simulink model "robotarm_NN"  (R2018b)
settings: Solver=FixedStepAuto  StartTime=0.0  StopTime=20  RelTol=1e-3  AbsTol=1e-6
undefined symbols (not defined in the file or in its folder): options
libraries: neural x132, simulink x2
(part 2 of 6)

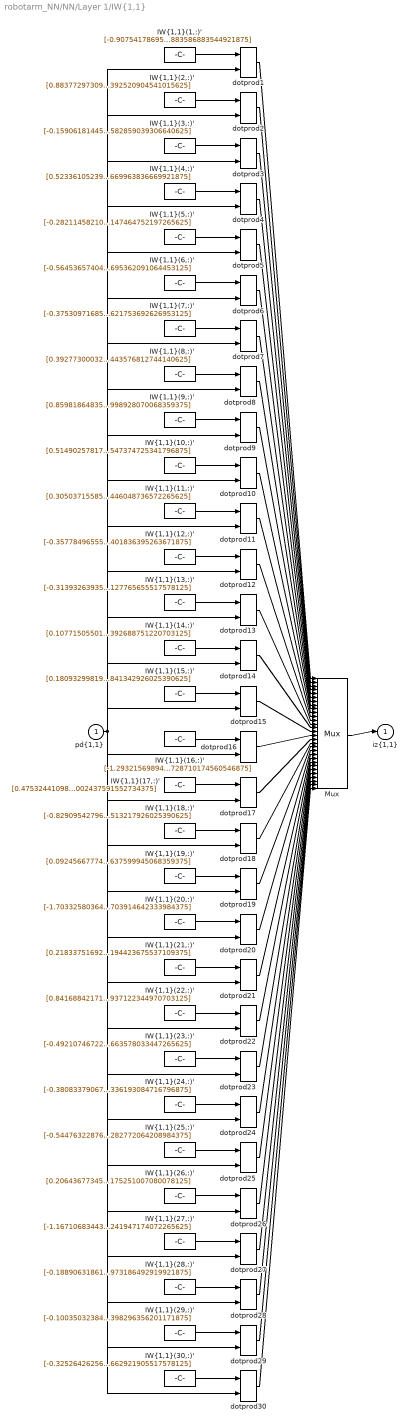
== system robotarm_NN/NN/Layer 1/IW{1,1} ==
  "pd{1,1}" : Inport  PortDimensions=10
      mask Display: e = 0.06;c1 = [120 230 180]/255;c2 = ([120 230 180]+0)/(256+128);c3 = ([120 230 180]+128)/(256+128);patch([0 1 1 0],[0 0 1 1],c1);patch([0 1 1 1-e 1-e 0+e],[0 0 1 1-e 0+e 0+e],c2);patch([0 0 1 1-e 0+e 0+e],[0 1 1 1-e 1-e 0+e],c3);plot([0 1 1 0 0],[0 0 1 1 0]);
  "IW{1,1}(1,:)'" : Constant  Value=[-0.90754178695281095823332861982635222375392913818359375;-0.742116818964511981704390564118511974811553955078125;0.412008312868980153265141552765271626412868499755859375;0.36505650495964692137107476810342632234096527099609375;0.8146542718376459379925336179439909756183624267578125;0.74217006261127071997663051661220379173755645751953125;-0.61338539843698958176076985182589851319789886474609375;-0.7369042666159348886623092766967602074146270751953125;0.67520008036012690855187656779889948666095733642578125;0.66999644798205515439093460372532717883586883544921875]
      mask Display: e = 0.06;c1 = [120 150 230]/255;c2 = ([120 150 230]+0)/383;c3 = ([120 150 230]+128)/383;patch([0 1 1 0],[0 0 1 1],c1);patch([0 1 1 1-e 1-e 0+e],[0 0 1 1-e 0+e 0+e],c2);patch([0 0 1 1-e 0+e 0+e],[0 1 1 1-e 1-e 0+e],c3);plot([0 1 1 0 0],[0 0 1 1 0]);disp('Weights');
  "IW{1,1}(10,:)'" : Constant  Value=[0.51490257817894524716706428080215118825435638427734375;-0.55689013510191454070508143558981828391551971435546875;-1.0160440906229057933529702495434321463108062744140625;0.833148456201297182843745758873410522937774658203125;0.2978923037071978807688310553203336894512176513671875;0.44937108713853712860242239912622608244419097900390625;-1.232430563498764453100875471136532723903656005859375;0.51275755356745766899706495678401552140712738037109375;0.271725160862764714142514321792987175285816192626953125;-0.256572494217802204996559112260001711547374725341796875]
      mask Display: e = 0.06;c1 = [120 150 230]/255;c2 = ([120 150 230]+0)/383;c3 = ([120 150 230]+128)/383;patch([0 1 1 0],[0 0 1 1],c1);patch([0 1 1 1-e 1-e 0+e],[0 0 1 1-e 0+e 0+e],c2);patch([0 0 1 1-e 0+e 0+e],[0 1 1 1-e 1-e 0+e],c3);plot([0 1 1 0 0],[0 0 1 1 0]);disp('Weights');
  "IW{1,1}(11,:)'" : Constant  Value=[0.305037155853193298060688221085001714527606964111328125;-0.2027495084904122613078669701280887238681316375732421875;0.36978378222056462742983740099589340388774871826171875;-0.197773141378723538164052797583281062543392181396484375;-0.9166473771667875691804283633246086537837982177734375;0.396221944755875465915551103535108268260955810546875;0.63562023332642991757523986962041817605495452880859375;-0.317476462047965368729052215712727047502994537353515625;-0.47855106483382947590854428199236281216144561767578125;-0.17691155876204567309883941561565734446048736572265625]
      mask Display: e = 0.06;c1 = [120 150 230]/255;c2 = ([120 150 230]+0)/383;c3 = ([120 150 230]+128)/383;patch([0 1 1 0],[0 0 1 1],c1);patch([0 1 1 1-e 1-e 0+e],[0 0 1 1-e 0+e 0+e],c2);patch([0 0 1 1-e 0+e 0+e],[0 1 1 1-e 1-e 0+e],c3);plot([0 1 1 0 0],[0 0 1 1 0]);disp('Weights');
  "IW{1,1}(12,:)'" : Constant  Value=[-0.357784965557944811820334507501684129238128662109375;0.055735883088791481065893407276234938763082027435302734375;-0.313420924791760924232875140660325996577739715576171875;0.208971447740384952407310947819496504962444305419921875;0.05285933764594109851575609582141623832285404205322265625;0.1769619850972858066118220676798955537378787994384765625;0.39701106906844174648796297333319671452045440673828125;-0.580802733316371888605544882011599838733673095703125;0.488751125745354231266759370555519126355648040771484375;0.286192921309179393318800066481344401836395263671875]
      mask Display: e = 0.06;c1 = [120 150 230]/255;c2 = ([120 150 230]+0)/383;c3 = ([120 150 230]+128)/383;patch([0 1 1 0],[0 0 1 1],c1);patch([0 1 1 1-e 1-e 0+e],[0 0 1 1-e 0+e 0+e],c2);patch([0 0 1 1-e 0+e 0+e],[0 1 1 1-e 1-e 0+e],c3);plot([0 1 1 0 0],[0 0 1 1 0]);disp('Weights');
  "IW{1,1}(13,:)'" : Constant  Value=[-0.313932639357311138450512544295634143054485321044921875;0.1727003133501055776033439315142459236085414886474609375;-0.449742884363723061103002009986084885895252227783203125;-0.899984540044212355525132807088084518909454345703125;0.62570865913053486107031631036079488694667816162109375;-1.2149239085840297658336339736706577241420745849609375;-0.562888595019426229981718279304914176464080810546875;0.1384465462583843731181332259438931941986083984375;-0.462843070858717509086233121706754900515079498291015625;0.09715649847031544716902118352663819678127765655517578125]
      mask Display: e = 0.06;c1 = [120 150 230]/255;c2 = ([120 150 230]+0)/383;c3 = ([120 150 230]+128)/383;patch([0 1 1 0],[0 0 1 1],c1);patch([0 1 1 1-e 1-e 0+e],[0 0 1 1-e 0+e 0+e],c2);patch([0 0 1 1-e 0+e 0+e],[0 1 1 1-e 1-e 0+e],c3);plot([0 1 1 0 0],[0 0 1 1 0]);disp('Weights');
  "IW{1,1}(14,:)'" : Constant  Value=[0.10771505501826938999698768384405411779880523681640625;-0.3394646908850085242903560356353409588336944580078125;-0.53916331936700834237541357651934958994388580322265625;0.78734972615334652967788997557363472878932952880859375;0.1999505506455650227781717376274173147976398468017578125;-0.033551712972406111390455407672561705112457275390625;-0.89834197551024230765648326269001699984073638916015625;0.726508718029837741170240406063385307788848876953125;-0.055448625277211886774875182481991942040622234344482421875;0.2113631602370545092828280075991642661392688751220703125]
      mask Display: e = 0.06;c1 = [120 150 230]/255;c2 = ([120 150 230]+0)/383;c3 = ([120 150 230]+128)/383;patch([0 1 1 0],[0 0 1 1],c1);patch([0 1 1 1-e 1-e 0+e],[0 0 1 1-e 0+e 0+e],c2);patch([0 0 1 1-e 0+e 0+e],[0 1 1 1-e 1-e 0+e],c3);plot([0 1 1 0 0],[0 0 1 1 0]);disp('Weights');
  "IW{1,1}(15,:)'" : Constant  Value=[0.180932998199578698450551428322796709835529327392578125;-0.4901383389807036916607785315136425197124481201171875;0.86034734548100078033172621871926821768283843994140625;-0.66432972863257921947166551035479642450809478759765625;-0.3365573093663172254963455998222343623638153076171875;0.85441020638785492025135681615211069583892822265625;0.453868542891665172067661160326679237186908721923828125;-0.88814808976047421307242757393396459519863128662109375;0.392618260181794909158270456828176975250244140625;0.429304143659537340571574759451323188841342926025390625]
      mask Display: e = 0.06;c1 = [120 150 230]/255;c2 = ([120 150 230]+0)/383;c3 = ([120 150 230]+128)/383;patch([0 1 1 0],[0 0 1 1],c1);patch([0 1 1 1-e 1-e 0+e],[0 0 1 1-e 0+e 0+e],c2);patch([0 0 1 1-e 0+e 0+e],[0 1 1 1-e 1-e 0+e],c3);plot([0 1 1 0 0],[0 0 1 1 0]);disp('Weights');
  "IW{1,1}(16,:)'" : Constant  Value=[-1.2932156989487475495792523361160419881343841552734375;0.2348824002906516328348374145207344554364681243896484375;1.22219610665761369006077075027860701084136962890625;0.06810109120647929448200130764234927482903003692626953125;0.330700925061075790001297036724281497299671173095703125;-0.59321813807871881518707368741161189973354339599609375;0.3290724853204503030923433470888994634151458740234375;1.352047501427814157892726143472827970981597900390625;0.11679471309927648425830426504035131074488162994384765625;1.070412264956114523073438249411992728710174560546875]
      mask Display: e = 0.06;c1 = [120 150 230]/255;c2 = ([120 150 230]+0)/383;c3 = ([120 150 230]+128)/383;patch([0 1 1 0],[0 0 1 1],c1);patch([0 1 1 1-e 1-e 0+e],[0 0 1 1-e 0+e 0+e],c2);patch([0 0 1 1-e 0+e 0+e],[0 1 1 1-e 1-e 0+e],c3);plot([0 1 1 0 0],[0 0 1 1 0]);disp('Weights');
  "IW{1,1}(17,:)'" : Constant  Value=[0.475324410980221545575119534987607039511203765869140625;-0.706642176870218907680509801139123737812042236328125;0.626780648758788583307932640309445559978485107421875;-0.53824722400187152704376103429240174591541290283203125;-0.1420312956212367583308520124774076975882053375244140625;1.4889718774801414813424571548239327967166900634765625;-1.0974261626859627138941277735284529626369476318359375;-0.047492401326013684859095320689448271878063678741455078125;0.6049041711880158711522881276323460042476654052734375;0.0666820294218544995512587547636940144002437591552734375]
      mask Display: e = 0.06;c1 = [120 150 230]/255;c2 = ([120 150 230]+0)/383;c3 = ([120 150 230]+128)/383;patch([0 1 1 0],[0 0 1 1],c1);patch([0 1 1 1-e 1-e 0+e],[0 0 1 1-e 0+e 0+e],c2);patch([0 0 1 1-e 0+e 0+e],[0 1 1 1-e 1-e 0+e],c3);plot([0 1 1 0 0],[0 0 1 1 0]);disp('Weights');
  "IW{1,1}(18,:)'" : Constant  Value=[-0.82909542796290913724277515939320437610149383544921875;0.357889890498670870666586552033550105988979339599609375;0.377881242025902286396643603438860736787319183349609375;-1.1818437177235503465766441877349279820919036865234375;0.89637578451523747258278262961539439857006072998046875;0.7278877221736512748151426421827636659145355224609375;-0.8064244092621748460913977396558038890361785888671875;-0.125054286779346213176467017547111026942729949951171875;-0.65982040286563348185921995536773465573787689208984375;-0.8101809081008151114389193025999702513217926025390625]
      mask Display: e = 0.06;c1 = [120 150 230]/255;c2 = ([120 150 230]+0)/383;c3 = ([120 150 230]+128)/383;patch([0 1 1 0],[0 0 1 1],c1);patch([0 1 1 1-e 1-e 0+e],[0 0 1 1-e 0+e 0+e],c2);patch([0 0 1 1-e 0+e 0+e],[0 1 1 1-e 1-e 0+e],c3);plot([0 1 1 0 0],[0 0 1 1 0]);disp('Weights');
  "IW{1,1}(19,:)'" : Constant  Value=[0.09245667774062486798936078002952854149043560028076171875;-0.36547098591766824515758571578771807253360748291015625;0.5826662519137666418345133934053592383861541748046875;0.5685848990998481067293823798536323010921478271484375;0.169176241475702815453274752144352532923221588134765625;-0.45304175453532125050770673624356277287006378173828125;0.182151688990629112563368607879965566098690032958984375;0.3263711021793713751293353197979740798473358154296875;-0.51320312083761010502058752535958774387836456298828125;-1.530053500052245052387434043339453637599945068359375]
      mask Display: e = 0.06;c1 = [120 150 230]/255;c2 = ([120 150 230]+0)/383;c3 = ([120 150 230]+128)/383;patch([0 1 1 0],[0 0 1 1],c1);patch([0 1 1 1-e 1-e 0+e],[0 0 1 1-e 0+e 0+e],c2);patch([0 0 1 1-e 0+e 0+e],[0 1 1 1-e 1-e 0+e],c3);plot([0 1 1 0 0],[0 0 1 1 0]);disp('Weights');
  "IW{1,1}(2,:)'" : Constant  Value=[0.88377297309429125871105270562111400067806243896484375;-0.138887088618623921743022719965665601193904876708984375;-0.202085156373757623970988106520962901413440704345703125;-0.368011816338925712432939008067478425800800323486328125;0.752272211114789257635493413545191287994384765625;-1.161956971024128204561520760762505233287811279296875;-0.06392607512588997786817657242863788269460201263427734375;0.368549590359761480851119586077402345836162567138671875;0.05283489042237192456763494874394382350146770477294921875;-1.0321689188508627044171817033202387392520904541015625]
      mask Display: e = 0.06;c1 = [120 150 230]/255;c2 = ([120 150 230]+0)/383;c3 = ([120 150 230]+128)/383;patch([0 1 1 0],[0 0 1 1],c1);patch([0 1 1 1-e 1-e 0+e],[0 0 1 1-e 0+e 0+e],c2);patch([0 0 1 1-e 0+e 0+e],[0 1 1 1-e 1-e 0+e],c3);plot([0 1 1 0 0],[0 0 1 1 0]);disp('Weights');
  "IW{1,1}(20,:)'" : Constant  Value=[-1.7033258036463692075557219141046516597270965576171875;1.0835398695150992853797333737020380795001983642578125;1.0886754741746316188510945721645839512348175048828125;0.1531937798604103562194467258450458757579326629638671875;-0.60410233591964590527112477502669207751750946044921875;1.174543327367428613428046446642838418483734130859375;0.6710480520276800309176223890972323715686798095703125;-0.397544452401657755213904010815895162522792816162109375;0.87980857575505588830111491915886290371417999267578125;0.93443898209996145709510528831742703914642333984375]
      mask Display: e = 0.06;c1 = [120 150 230]/255;c2 = ([120 150 230]+0)/383;c3 = ([120 150 230]+128)/383;patch([0 1 1 0],[0 0 1 1],c1);patch([0 1 1 1-e 1-e 0+e],[0 0 1 1-e 0+e 0+e],c2);patch([0 0 1 1-e 0+e 0+e],[0 1 1 1-e 1-e 0+e],c3);plot([0 1 1 0 0],[0 0 1 1 0]);disp('Weights');
  "IW{1,1}(21,:)'" : Constant  Value=[0.2183375169279730132476657900042482651770114898681640625;1.0295477724541246544731620815582573413848876953125;0.57849360328365329042554776606266386806964874267578125;0.92788643865950337641379519482143223285675048828125;0.08067220756117073066082667764931102283298969268798828125;-0.301239654696074221629231715269270353019237518310546875;-0.096490564950137691635490000408026389777660369873046875;0.59347250715547839039487598711275495588779449462890625;0.1565068836928611151204648876955616287887096405029296875;-0.328401760290170263711928555494523607194423675537109375]
      mask Display: e = 0.06;c1 = [120 150 230]/255;c2 = ([120 150 230]+0)/383;c3 = ([120 150 230]+128)/383;patch([0 1 1 0],[0 0 1 1],c1);patch([0 1 1 1-e 1-e 0+e],[0 0 1 1-e 0+e 0+e],c2);patch([0 0 1 1-e 0+e 0+e],[0 1 1 1-e 1-e 0+e],c3);plot([0 1 1 0 0],[0 0 1 1 0]);disp('Weights');
  "IW{1,1}(22,:)'" : Constant  Value=[0.84168842171868629709052811449510045349597930908203125;-0.32274305996753993586168007823289372026920318603515625;0.50011509190905112376412944286130368709564208984375;0.41243847101874842042690261223469860851764678955078125;0.408931498274886118249327182638808153569698333740234375;-0.449185026625067151950787547320942394435405731201171875;-0.28385476516801855240146323922090232372283935546875;1.24608929925965838947377051226794719696044921875;-0.50416494519493182391300933886668644845485687255859375;0.289501186146771172236213942596805281937122344970703125]
      mask Display: e = 0.06;c1 = [120 150 230]/255;c2 = ([120 150 230]+0)/383;c3 = ([120 150 230]+128)/383;patch([0 1 1 0],[0 0 1 1],c1);patch([0 1 1 1-e 1-e 0+e],[0 0 1 1-e 0+e 0+e],c2);patch([0 0 1 1-e 0+e 0+e],[0 1 1 1-e 1-e 0+e],c3);plot([0 1 1 0 0],[0 0 1 1 0]);disp('Weights');
  "IW{1,1}(23,:)'" : Constant  Value=[-0.492107467227739459048052594880573451519012451171875;-0.286959259625639007129649371563573367893695831298828125;0.289706447444466996810064074452384375035762786865234375;0.33083963330364529742411150436964817345142364501953125;1.4243534128318771081467275507748126983642578125;-1.1893652306332975765457149464054964482784271240234375;-0.2119553555973208158746956542017869651317596435546875;0.00113831771756360057047674505525947097339667379856109619140625;0.4705420118572136711776465745060704648494720458984375;0.2211802845954346230517018057071254588663578033447265625]
      mask Display: e = 0.06;c1 = [120 150 230]/255;c2 = ([120 150 230]+0)/383;c3 = ([120 150 230]+128)/383;patch([0 1 1 0],[0 0 1 1],c1);patch([0 1 1 1-e 1-e 0+e],[0 0 1 1-e 0+e 0+e],c2);patch([0 0 1 1-e 0+e 0+e],[0 1 1 1-e 1-e 0+e],c3);plot([0 1 1 0 0],[0 0 1 1 0]);disp('Weights');
  "IW{1,1}(24,:)'" : Constant  Value=[-0.38083379067342348900382376086781732738018035888671875;0.53926105013783975916652480009361170232295989990234375;-0.017681855452514085025317314148196601308882236480712890625;0.09794479586322714370627551261350163258612155914306640625;0.4458190384504678860366766457445919513702392578125;-0.5133283534781523105294809283805079758167266845703125;0.2332310287153489536393635717104189097881317138671875;-0.08687379869584781200142487023185822181403636932373046875;-0.2668001734199625385457466109073720872402191162109375;-0.6722409363213994737407119828276336193084716796875]
      mask Display: e = 0.06;c1 = [120 150 230]/255;c2 = ([120 150 230]+0)/383;c3 = ([120 150 230]+128)/383;patch([0 1 1 0],[0 0 1 1],c1);patch([0 1 1 1-e 1-e 0+e],[0 0 1 1-e 0+e 0+e],c2);patch([0 0 1 1-e 0+e 0+e],[0 1 1 1-e 1-e 0+e],c3);plot([0 1 1 0 0],[0 0 1 1 0]);disp('Weights');
  "IW{1,1}(25,:)'" : Constant  Value=[-0.544763228766832252603080632979981601238250732421875;1.025583716006354340066764052608050405979156494140625;-0.3909767965032313608020331230363808572292327880859375;0.175392199570192641733257232772302813827991485595703125;0.1312694927322486104781518179152044467628002166748046875;-0.29628612774353968450924412536551244556903839111328125;0.627045442519258866553855114034377038478851318359375;-0.494734533770225859417024594222311861813068389892578125;-0.1709269662642663167861911688305553980171680450439453125;-0.712029567731066403979411916225217282772064208984375]
      mask Display: e = 0.06;c1 = [120 150 230]/255;c2 = ([120 150 230]+0)/383;c3 = ([120 150 230]+128)/383;patch([0 1 1 0],[0 0 1 1],c1);patch([0 1 1 1-e 1-e 0+e],[0 0 1 1-e 0+e 0+e],c2);patch([0 0 1 1-e 0+e 0+e],[0 1 1 1-e 1-e 0+e],c3);plot([0 1 1 0 0],[0 0 1 1 0]);disp('Weights');
  "IW{1,1}(26,:)'" : Constant  Value=[0.2064367734516230068475550751827540807425975799560546875;-0.52171204350552746742408771751797758042812347412109375;0.465670328613799366923586831035208888351917266845703125;-0.6770397893822426294008209879393689334392547607421875;-0.007157899521067303573451656717452351585961878299713134765625;0.53060398438798983544728571359883062541484832763671875;-0.471639027281536282742990806582383811473846435546875;0.1027639569281287579283201694124727509915828704833984375;-1.2114700866999077444319254936999641358852386474609375;-0.1727137841860635625312880847559426911175251007080078125]
      mask Display: e = 0.06;c1 = [120 150 230]/255;c2 = ([120 150 230]+0)/383;c3 = ([120 150 230]+128)/383;patch([0 1 1 0],[0 0 1 1],c1);patch([0 1 1 1-e 1-e 0+e],[0 0 1 1-e 0+e 0+e],c2);patch([0 0 1 1-e 0+e 0+e],[0 1 1 1-e 1-e 0+e],c3);plot([0 1 1 0 0],[0 0 1 1 0]);disp('Weights');
  "IW{1,1}(27,:)'" : Constant  Value=[-1.167106834431565598464430877356790006160736083984375;0.437522360025288048479552571734529919922351837158203125;0.300094058637896343721962466588593088090419769287109375;0.83712371673845831221427715718164108693599700927734375;0.35996393405444992996677910923608578741550445556640625;0.91710359831558008192331499230931513011455535888671875;-0.018912989989779908917011397306850994937121868133544921875;-0.34942573076748117966161544245551340281963348388671875;-0.10919776267308552164525536909422953613102436065673828125;0.1766103783628904244640267506838426925241947174072265625]
      mask Display: e = 0.06;c1 = [120 150 230]/255;c2 = ([120 150 230]+0)/383;c3 = ([120 150 230]+128)/383;patch([0 1 1 0],[0 0 1 1],c1);patch([0 1 1 1-e 1-e 0+e],[0 0 1 1-e 0+e 0+e],c2);patch([0 0 1 1-e 0+e 0+e],[0 1 1 1-e 1-e 0+e],c3);plot([0 1 1 0 0],[0 0 1 1 0]);disp('Weights');
  "IW{1,1}(28,:)'" : Constant  Value=[-0.1889063186112509284964033895448665134608745574951171875;-0.10349718007234449956843747031598468311131000518798828125;-0.6004000904711210839792556726024486124515533447265625;-0.070715733660242252600625079139717854559421539306640625;0.69180246406658396640665387167246080935001373291015625;0.25852977217707351353936928717303089797496795654296875;0.6492678655596717529618899789056740701198577880859375;-0.82723962588871902124054713567602448165416717529296875;0.75029201855868965509444024064578115940093994140625;0.54667245330583547069380756511236540973186492919921875]
      mask Display: e = 0.06;c1 = [120 150 230]/255;c2 = ([120 150 230]+0)/383;c3 = ([120 150 230]+128)/383;patch([0 1 1 0],[0 0 1 1],c1);patch([0 1 1 1-e 1-e 0+e],[0 0 1 1-e 0+e 0+e],c2);patch([0 0 1 1-e 0+e 0+e],[0 1 1 1-e 1-e 0+e],c3);plot([0 1 1 0 0],[0 0 1 1 0]);disp('Weights');
  "IW{1,1}(29,:)'" : Constant  Value=[-0.10035032384524221471533422800348489545285701751708984375;0.026152669218288786268100665211022715084254741668701171875;-0.1635053996569839351860053966447594575583934783935546875;-0.11170709510527747354569072513186256401240825653076171875;-0.46670879047304481002100828845868818461894989013671875;-0.314925914363283820929240164332441054284572601318359375;0.76961274436453230851640228138421662151813507080078125;-0.41880061878503482830637949518859386444091796875;-0.445818816682043650434508208491024561226367950439453125;-1.242321292491154860471169740776531398296356201171875]
      mask Display: e = 0.06;c1 = [120 150 230]/255;c2 = ([120 150 230]+0)/383;c3 = ([120 150 230]+128)/383;patch([0 1 1 0],[0 0 1 1],c1);patch([0 1 1 1-e 1-e 0+e],[0 0 1 1-e 0+e 0+e],c2);patch([0 0 1 1-e 0+e 0+e],[0 1 1 1-e 1-e 0+e],c3);plot([0 1 1 0 0],[0 0 1 1 0]);disp('Weights');
  "IW{1,1}(3,:)'" : Constant  Value=[-0.1590618144508099962575187191760051064193248748779296875;0.2389546407019083329448250196946901269257068634033203125;0.7336894557773774305786673721740953624248504638671875;-0.54901256230777539801835018806741572916507720947265625;0.34600912765164881790269646444357931613922119140625;-0.78333308706623971939819739418453536927700042724609375;-0.33015710310938717331197267412790097296237945556640625;-0.114983759636541449378199786224286071956157684326171875;0.28177934529329007329323530939291231334209442138671875;-0.8686981054090241460841070875176228582859039306640625]
      mask Display: e = 0.06;c1 = [120 150 230]/255;c2 = ([120 150 230]+0)/383;c3 = ([120 150 230]+128)/383;patch([0 1 1 0],[0 0 1 1],c1);patch([0 1 1 1-e 1-e 0+e],[0 0 1 1-e 0+e 0+e],c2);patch([0 0 1 1-e 0+e 0+e],[0 1 1 1-e 1-e 0+e],c3);plot([0 1 1 0 0],[0 0 1 1 0]);disp('Weights');
  "IW{1,1}(30,:)'" : Constant  Value=[-0.325264262569930406865381655734381638467311859130859375;0.168411484861244797883728097076527774333953857421875;0.66135120865834673420380340758129023015499114990234375;0.67796924186734142114829637648654170334339141845703125;0.52291844981728130559162082136026583611965179443359375;-0.23878341865806873567379398082266561686992645263671875;-0.180229906390271976679429144496680237352848052978515625;0.38130978888805711068954451548052020370960235595703125;-0.5001462112598222820025739565608091652393341064453125;-0.477555210350722791901034725015051662921905517578125]
      mask Display: e = 0.06;c1 = [120 150 230]/255;c2 = ([120 150 230]+0)/383;c3 = ([120 150 230]+128)/383;patch([0 1 1 0],[0 0 1 1],c1);patch([0 1 1 1-e 1-e 0+e],[0 0 1 1-e 0+e 0+e],c2);patch([0 0 1 1-e 0+e 0+e],[0 1 1 1-e 1-e 0+e],c3);plot([0 1 1 0 0],[0 0 1 1 0]);disp('Weights');
  "IW{1,1}(4,:)'" : Constant  Value=[0.52336105239007391087824316855403594672679901123046875;-0.499597767422709948537118407330126501619815826416015625;-0.8930416526326643289479534359998069703578948974609375;0.0672058413510440988414273988382774405181407928466796875;1.0680749238524327449084694308112375438213348388671875;0.2441220891907126266939798142630024813115596771240234375;0.11972634969445440644708611444002599455416202545166015625;-0.6430882075409198872506522093317471444606781005859375;-0.100144167413062368243714672644273377954959869384765625;-0.8777661451407119397316591857816092669963836669921875]
      mask Display: e = 0.06;c1 = [120 150 230]/255;c2 = ([120 150 230]+0)/383;c3 = ([120 150 230]+128)/383;patch([0 1 1 0],[0 0 1 1],c1);patch([0 1 1 1-e 1-e 0+e],[0 0 1 1-e 0+e 0+e],c2);patch([0 0 1 1-e 0+e 0+e],[0 1 1 1-e 1-e 0+e],c3);plot([0 1 1 0 0],[0 0 1 1 0]);disp('Weights');
  "IW{1,1}(5,:)'" : Constant  Value=[-0.28211458210886830588748352965922094881534576416015625;-0.53925926187068962125437110444181598722934722900390625;-0.89484118217413011198146932656527496874332427978515625;0.0032860484087374364388367542488822437007911503314971923828125;-0.144786966237127223688929689160431735217571258544921875;0.437316110674828895099608416785486042499542236328125;-0.68593572751167564138796706174616701900959014892578125;-0.409907519252667551512558929971419274806976318359375;-0.7550413527152251003116134597803466022014617919921875;-0.434547708115560260555554350503371097147464752197265625]
      mask Display: e = 0.06;c1 = [120 150 230]/255;c2 = ([120 150 230]+0)/383;c3 = ([120 150 230]+128)/383;patch([0 1 1 0],[0 0 1 1],c1);patch([0 1 1 1-e 1-e 0+e],[0 0 1 1-e 0+e 0+e],c2);patch([0 0 1 1-e 0+e 0+e],[0 1 1 1-e 1-e 0+e],c3);plot([0 1 1 0 0],[0 0 1 1 0]);disp('Weights');
  "IW{1,1}(6,:)'" : Constant  Value=[-0.5645365740454020286875902456813491880893707275390625;0.27979648554409364269446314210654236376285552978515625;0.5671404224277256655994960965472273528575897216796875;-0.85546822259963894996559474748210050165653228759765625;-0.37748122962170660432690283414558507502079010009765625;0.1993402318735925937698283405552501790225505828857421875;0.1647171497075255730546672339187352918088436126708984375;-0.7639067868727680288287729126750491559505462646484375;0.51699550360281720795541104962467215955257415771484375;0.8014205434996046761852994677610695362091064453125]
      mask Display: e = 0.06;c1 = [120 150 230]/255;c2 = ([120 150 230]+0)/383;c3 = ([120 150 230]+128)/383;patch([0 1 1 0],[0 0 1 1],c1);patch([0 1 1 1-e 1-e 0+e],[0 0 1 1-e 0+e 0+e],c2);patch([0 0 1 1-e 0+e 0+e],[0 1 1 1-e 1-e 0+e],c3);plot([0 1 1 0 0],[0 0 1 1 0]);disp('Weights');
  "IW{1,1}(7,:)'" : Constant  Value=[-0.375309716854690555987161815210129134356975555419921875;-0.4260242744010949156319156827521510422229766845703125;-0.0716848811463306201385847771234693937003612518310546875;-0.60115326778078748137801312623196281492710113525390625;0.836366105265711201610656644334085285663604736328125;0.79509146449892842412054960732348263263702392578125;-0.9889721466686498541065475365030579268932342529296875;0.1938843954843518790909229210228659212589263916015625;-1.3982580469026471003957112770876847207546234130859375;-0.68777467007829617973158065069583244621753692626953125]
      mask Display: e = 0.06;c1 = [120 150 230]/255;c2 = ([120 150 230]+0)/383;c3 = ([120 150 230]+128)/383;patch([0 1 1 0],[0 0 1 1],c1);patch([0 1 1 1-e 1-e 0+e],[0 0 1 1-e 0+e 0+e],c2);patch([0 0 1 1-e 0+e 0+e],[0 1 1 1-e 1-e 0+e],c3);plot([0 1 1 0 0],[0 0 1 1 0]);disp('Weights');
  "IW{1,1}(8,:)'" : Constant  Value=[0.392773000321874510287756265825009904801845550537109375;-0.8587381173702055559004975293646566569805145263671875;0.134476894032145521951093769530416466295719146728515625;-0.422620695609751795274178221006877720355987548828125;0.09253882802590761291749998918021447025239467620849609375;0.60881467657779475555201997849508188664913177490234375;-1.053175297640367436002861722954548895359039306640625;-0.2422690683791939025848449773548054508864879608154296875;0.484610135172203915221444958660867996513843536376953125;0.6026905823252735050488126944401301443576812744140625]
      mask Display: e = 0.06;c1 = [120 150 230]/255;c2 = ([120 150 230]+0)/383;c3 = ([120 150 230]+128)/383;patch([0 1 1 0],[0 0 1 1],c1);patch([0 1 1 1-e 1-e 0+e],[0 0 1 1-e 0+e 0+e],c2);patch([0 0 1 1-e 0+e 0+e],[0 1 1 1-e 1-e 0+e],c3);plot([0 1 1 0 0],[0 0 1 1 0]);disp('Weights');
  "IW{1,1}(9,:)'" : Constant  Value=[0.85981864835182619799525127746164798736572265625;-1.00836295042848878011909619090147316455841064453125;-0.58199389552080538212663896047160960733890533447265625;-0.10519245397793637597505522762730834074318408966064453125;0.17009317654878197689782837187522090971469879150390625;0.1694579593970052255880176517166546545922756195068359375;0.63984435026716457439732721468317322432994842529296875;0.7195856291378850411177836576825939118862152099609375;-0.1833123682309809598933725283131934702396392822265625;-0.606197422257591878036464549950323998928070068359375]
      mask Display: e = 0.06;c1 = [120 150 230]/255;c2 = ([120 150 230]+0)/383;c3 = ([120 150 230]+128)/383;patch([0 1 1 0],[0 0 1 1],c1);patch([0 1 1 1-e 1-e 0+e],[0 0 1 1-e 0+e 0+e],c2);patch([0 0 1 1-e 0+e 0+e],[0 1 1 1-e 1-e 0+e],c3);plot([0 1 1 0 0],[0 0 1 1 0]);disp('Weights');
  Mux : Mux  Inputs=30
      mask Display: e = 0.06;c1 = [120 150 230]/255;c2 = ([120 150 230]+0)/383;c3 = ([120 150 230]+128)/383;patch([0 1 1 0],[0 0 1 1],c1);patch([0 1 1 1-e 1-e 0+e],[0 0 1 1-e 0+e 0+e],c2);patch([0 0 1 1-e 0+e 0+e],[0 1 1 1-e 1-e 0+e],c3);plot([0 1 1 0 0],[0 0 1 1 0]);disp('Mux');
  dotprod{1..30} (30 alike) : neural/Weight Functions/dotprod
  "iz{1,1}" : Outport
      mask Display: e = 0.06;c1 = [120 230 180]/255;c2 = ([120 230 180]+0)/(256+128);c3 = ([120 230 180]+128)/(256+128);patch([0 1 1 0],[0 0 1 1],c1);patch([0 1 1 1-e 1-e 0+e],[0 0 1 1-e 0+e 0+e],c2);patch([0 0 1 1-e 0+e 0+e],[0 1 1 1-e 1-e 0+e],c3);plot([0 1 1 0 0],[0 0 1 1 0]);
  wires:
  "IW{1,1}(1,:)'"/1 -> dotprod1/1
  "pd{1,1}"/1 -> dotprod1/2, dotprod2/2, dotprod3/2, dotprod4/2, dotprod5/2, dotprod6/2, dotprod7/2, dotprod8/2, dotprod9/2, dotprod10/2, dotprod11/2, dotprod12/2, dotprod13/2, dotprod14/2, dotprod15/2, dotprod16/2, dotprod17/2, dotprod18/2, dotprod19/2, dotprod20/2, dotprod21/2, dotprod22/2, dotprod23/2, dotprod24/2, dotprod25/2, dotprod26/2, dotprod27/2, dotprod28/2, dotprod29/2, dotprod30/2
  dotprod1/1 -> Mux/1
  "IW{1,1}(2,:)'"/1 -> dotprod2/1
  dotprod2/1 -> Mux/2
  "IW{1,1}(3,:)'"/1 -> dotprod3/1
  dotprod3/1 -> Mux/3
  "IW{1,1}(4,:)'"/1 -> dotprod4/1
  dotprod4/1 -> Mux/4
  "IW{1,1}(5,:)'"/1 -> dotprod5/1
  dotprod5/1 -> Mux/5
  "IW{1,1}(6,:)'"/1 -> dotprod6/1
  dotprod6/1 -> Mux/6
  "IW{1,1}(7,:)'"/1 -> dotprod7/1
  dotprod7/1 -> Mux/7
  "IW{1,1}(8,:)'"/1 -> dotprod8/1
  dotprod8/1 -> Mux/8
  "IW{1,1}(9,:)'"/1 -> dotprod9/1
  dotprod9/1 -> Mux/9
  "IW{1,1}(10,:)'"/1 -> dotprod10/1
  dotprod10/1 -> Mux/10
  "IW{1,1}(11,:)'"/1 -> dotprod11/1
  dotprod11/1 -> Mux/11
  "IW{1,1}(12,:)'"/1 -> dotprod12/1
  dotprod12/1 -> Mux/12
  "IW{1,1}(13,:)'"/1 -> dotprod13/1
  dotprod13/1 -> Mux/13
  "IW{1,1}(14,:)'"/1 -> dotprod14/1
  dotprod14/1 -> Mux/14
  "IW{1,1}(15,:)'"/1 -> dotprod15/1
  dotprod15/1 -> Mux/15
  "IW{1,1}(16,:)'"/1 -> dotprod16/1
  dotprod16/1 -> Mux/16
  "IW{1,1}(17,:)'"/1 -> dotprod17/1
  dotprod17/1 -> Mux/17
  "IW{1,1}(18,:)'"/1 -> dotprod18/1
  dotprod18/1 -> Mux/18
  "IW{1,1}(19,:)'"/1 -> dotprod19/1
  dotprod19/1 -> Mux/19
  "IW{1,1}(20,:)'"/1 -> dotprod20/1
  dotprod20/1 -> Mux/20
  "IW{1,1}(21,:)'"/1 -> dotprod21/1
  dotprod21/1 -> Mux/21
  "IW{1,1}(22,:)'"/1 -> dotprod22/1
  dotprod22/1 -> Mux/22
  "IW{1,1}(23,:)'"/1 -> dotprod23/1
  dotprod23/1 -> Mux/23
  "IW{1,1}(24,:)'"/1 -> dotprod24/1
  dotprod24/1 -> Mux/24
  "IW{1,1}(25,:)'"/1 -> dotprod25/1
  dotprod25/1 -> Mux/25
  "IW{1,1}(26,:)'"/1 -> dotprod26/1
  dotprod26/1 -> Mux/26
  "IW{1,1}(27,:)'"/1 -> dotprod27/1
  dotprod27/1 -> Mux/27
  "IW{1,1}(28,:)'"/1 -> dotprod28/1
  dotprod28/1 -> Mux/28
  "IW{1,1}(29,:)'"/1 -> dotprod29/1
  dotprod29/1 -> Mux/29
  "IW{1,1}(30,:)'"/1 -> dotprod30/1
  dotprod30/1 -> Mux/30
  Mux/1 -> "iz{1,1}"/1

== system robotarm_NN/NN/Layer 2/Delays 1 ==
  "p{2}" : Inport  PortDimensions=30
      mask Display: e = 0.06;c1 = [120 230 180]/255;c2 = ([120 230 180]+0)/(256+128);c3 = ([120 230 180]+128)/(256+128);patch([0 1 1 0],[0 0 1 1],c1);patch([0 1 1 1-e 1-e 0+e],[0 0 1 1-e 0+e 0+e],c2);patch([0 0 1 1-e 0+e 0+e],[0 1 1 1-e 1-e 0+e],c3);plot([0 1 1 0 0],[0 0 1 1 0]);
  mux : Mux  Inputs=1
      mask Display: e = 0.06;c1 = [120 150 230]/255;c2 = ([120 150 230]+0)/383;c3 = ([120 150 230]+128)/383;patch([0 1 1 0],[0 0 1 1],c1);patch([0 1 1 1-e 1-e 0+e],[0 0 1 1-e 0+e 0+e],c2);patch([0 0 1 1-e 0+e 0+e],[0 1 1 1-e 1-e 0+e],c3);plot([0 1 1 0 0],[0 0 1 1 0]);disp('Mux')
  "pd{2,1}" : Outport
      mask Display: e = 0.06;c1 = [120 230 180]/255;c2 = ([120 230 180]+0)/(256+128);c3 = ([120 230 180]+128)/(256+128);patch([0 1 1 0],[0 0 1 1],c1);patch([0 1 1 1-e 1-e 0+e],[0 0 1 1-e 0+e 0+e],c2);patch([0 0 1 1-e 0+e 0+e],[0 1 1 1-e 1-e 0+e],c3);plot([0 1 1 0 0],[0 0 1 1 0]);
  wires:
  "p{2}"/1 -> mux/1
  mux/1 -> "pd{2,1}"/1
